simulink model "ExtDem_SelectParameter"  (R2016b)
settings: configuration reference "CodeGenConfigSet" (kept outside this file)
values from neighbouring files (symbols this model uses):
  ExtDem_facFdbk_CUR = Calibration.Parameter    [init_ExtDem_SelectParameter.m]
  ExtDem_facFdbk_CURX = Calibration.Parameter    [init_ExtDem_SelectParameter.m]
  ExtDem_facFdbkLimit_C = Calibration.Parameter    [init_ExtDem_SelectParameter.m]
  ExtDem_facFdbkParSet0_C = Calibration.Parameter    [init_ExtDem_SelectParameter.m]
  ExtDem_facFdbkParSet1_C = Calibration.Parameter    [init_ExtDem_SelectParameter.m]
  ExtDem_facFdbkParSet2_C = Calibration.Parameter    [init_ExtDem_SelectParameter.m]
  ExtDem_facFdbkParSet3_C = Calibration.Parameter    [init_ExtDem_SelectParameter.m]
  ExtDem_facFdbkParSet4_C = Calibration.Parameter    [init_ExtDem_SelectParameter.m]
  ExtDem_facFdbkParSet5_C = Calibration.Parameter    [init_ExtDem_SelectParameter.m]
  ExtDem_facFdbkParSet6_C = Calibration.Parameter    [init_ExtDem_SelectParameter.m]
  ExtDem_facFdbkParSet7_C = Calibration.Parameter    [init_ExtDem_SelectParameter.m]
  ExtDem_facNAvrgPT1CorFac_C = Calibration.Parameter    [init_ExtDem_SelectParameter.m]
  ExtDem_facTrqPT1CorFac_C = Calibration.Parameter    [init_ExtDem_SelectParameter.m]
  ExtDem_KiCorTempFac_MAP = Calibration.Parameter    [init_ExtDem_SelectParameter.m]
  ExtDem_KiCorTempFac_MAPX = Calibration.Parameter    [init_ExtDem_SelectParameter.m]
  ExtDem_KiCorTempFac_MAPY = Calibration.Parameter    [init_ExtDem_SelectParameter.m]
  ExtDem_KiCorTrqFac_MAP = Calibration.Parameter    [init_ExtDem_SelectParameter.m]
  ExtDem_KiCorTrqFac_MAPX = Calibration.Parameter    [init_ExtDem_SelectParameter.m]
  ExtDem_KiCorTrqFac_MAPY = Calibration.Parameter    [init_ExtDem_SelectParameter.m]
  ExtDem_KpCorTempFac_MAP = Calibration.Parameter    [init_ExtDem_SelectParameter.m]
  ExtDem_KpCorTempFac_MAPX = Calibration.Parameter    [init_ExtDem_SelectParameter.m]
  ExtDem_KpCorTempFac_MAPY = Calibration.Parameter    [init_ExtDem_SelectParameter.m]
  ExtDem_KpCorTrqFac_MAP = Calibration.Parameter    [init_ExtDem_SelectParameter.m]
  ExtDem_KpCorTrqFac_MAPX = Calibration.Parameter    [init_ExtDem_SelectParameter.m]
  ExtDem_KpCorTrqFac_MAPY = Calibration.Parameter    [init_ExtDem_SelectParameter.m]
  ExtDem_Par0Cfg_C = Calibration.Parameter    [init_ExtDem_SelectParameter.m]
  ExtDem_Par0dnAccLim_C = Calibration.Parameter    [init_ExtDem_SelectParameter.m]
  ExtDem_Par0dnDeclLim_C = Calibration.Parameter    [init_ExtDem_SelectParameter.m]
  ExtDem_Par0dnDeclLimBrk_C = Calibration.Parameter    [init_ExtDem_SelectParameter.m]
  ExtDem_Par0FacFdbkTrqLosHi_C = Calibration.Parameter    [init_ExtDem_SelectParameter.m]
  ExtDem_Par0FacFdbkTrqLosLo_C = Calibration.Parameter    [init_ExtDem_SelectParameter.m]
  ExtDem_Par0IKi_C = Calibration.Parameter    [init_ExtDem_SelectParameter.m]
  ExtDem_Par0IKiNeg_C = Calibration.Parameter    [init_ExtDem_SelectParameter.m]
  ExtDem_Par0IKiPos_C = Calibration.Parameter    [init_ExtDem_SelectParameter.m]
  ExtDem_Par0InrtVeh_C = Calibration.Parameter    [init_ExtDem_SelectParameter.m]
  ExtDem_Par0nIWinNeg_C = Calibration.Parameter    [init_ExtDem_SelectParameter.m]
  ExtDem_Par0nIWinPos_C = Calibration.Parameter    [init_ExtDem_SelectParameter.m]
  ExtDem_Par0nPWinNeg_C = Calibration.Parameter    [init_ExtDem_SelectParameter.m]
  ExtDem_Par0nPWinPos_C = Calibration.Parameter    [init_ExtDem_SelectParameter.m]
  ExtDem_Par0PKp_C = Calibration.Parameter    [init_ExtDem_SelectParameter.m]
  ExtDem_Par0PKpNeg_C = Calibration.Parameter    [init_ExtDem_SelectParameter.m]
  ExtDem_Par0PKpPos_C = Calibration.Parameter    [init_ExtDem_SelectParameter.m]
  ExtDem_Par0TiFltTrqLosEst_C = Calibration.Parameter    [init_ExtDem_SelectParameter.m]
  ExtDem_Par1Cfg_C = Calibration.Parameter    [init_ExtDem_SelectParameter.m]
  ExtDem_Par1dnAccLim_C = Calibration.Parameter    [init_ExtDem_SelectParameter.m]
  ExtDem_Par1dnDeclLim_C = Calibration.Parameter    [init_ExtDem_SelectParameter.m]
  ExtDem_Par1dnDeclLimBrk_C = Calibration.Parameter    [init_ExtDem_SelectParameter.m]
  ExtDem_Par1FacFdbkTrqLosHi_C = Calibration.Parameter    [init_ExtDem_SelectParameter.m]
  ExtDem_Par1FacFdbkTrqLosLo_C = Calibration.Parameter    [init_ExtDem_SelectParameter.m]
  ExtDem_Par1IKi_C = Calibration.Parameter    [init_ExtDem_SelectParameter.m]
  ExtDem_Par1IKiNeg_C = Calibration.Parameter    [init_ExtDem_SelectParameter.m]
  ExtDem_Par1IKiPos_C = Calibration.Parameter    [init_ExtDem_SelectParameter.m]
  ExtDem_Par1InrtVeh_C = Calibration.Parameter    [init_ExtDem_SelectParameter.m]
  ExtDem_Par1nIWinNeg_C = Calibration.Parameter    [init_ExtDem_SelectParameter.m]
  ExtDem_Par1nIWinPos_C = Calibration.Parameter    [init_ExtDem_SelectParameter.m]
  ExtDem_Par1nPWinNeg_C = Calibration.Parameter    [init_ExtDem_SelectParameter.m]
  ExtDem_Par1nPWinPos_C = Calibration.Parameter    [init_ExtDem_SelectParameter.m]
  ExtDem_Par1PKp_C = Calibration.Parameter    [init_ExtDem_SelectParameter.m]
  ExtDem_Par1PKpNeg_C = Calibration.Parameter    [init_ExtDem_SelectParameter.m]
  ExtDem_Par1PKpPos_C = Calibration.Parameter    [init_ExtDem_SelectParameter.m]
  ExtDem_Par1TiFltTrqLosEst_C = Calibration.Parameter    [init_ExtDem_SelectParameter.m]
  ExtDem_Par2Cfg_C = Calibration.Parameter    [init_ExtDem_SelectParameter.m]
  ExtDem_Par2dnAccLim_C = Calibration.Parameter    [init_ExtDem_SelectParameter.m]
  ExtDem_Par2dnDeclLim_C = Calibration.Parameter    [init_ExtDem_SelectParameter.m]
  ExtDem_Par2dnDeclLimBrk_C = Calibration.Parameter    [init_ExtDem_SelectParameter.m]
  ExtDem_Par2FacFdbkTrqLosHi_C = Calibration.Parameter    [init_ExtDem_SelectParameter.m]
  ExtDem_Par2FacFdbkTrqLosLo_C = Calibration.Parameter    [init_ExtDem_SelectParameter.m]
  ExtDem_Par2IKi_C = Calibration.Parameter    [init_ExtDem_SelectParameter.m]
  ExtDem_Par2IKiNeg_C = Calibration.Parameter    [init_ExtDem_SelectParameter.m]
  ExtDem_Par2IKiPos_C = Calibration.Parameter    [init_ExtDem_SelectParameter.m]
  ExtDem_Par2InrtVeh_C = Calibration.Parameter    [init_ExtDem_SelectParameter.m]
  ExtDem_Par2nIWinNeg_C = Calibration.Parameter    [init_ExtDem_SelectParameter.m]
  ExtDem_Par2nIWinPos_C = Calibration.Parameter    [init_ExtDem_SelectParameter.m]
  ExtDem_Par2nPWinNeg_C = Calibration.Parameter    [init_ExtDem_SelectParameter.m]
  ExtDem_Par2nPWinPos_C = Calibration.Parameter    [init_ExtDem_SelectParameter.m]
  ExtDem_Par2PKp_C = Calibration.Parameter    [init_ExtDem_SelectParameter.m]
  ExtDem_Par2PKpNeg_C = Calibration.Parameter    [init_ExtDem_SelectParameter.m]
  ExtDem_Par2PKpPos_C = Calibration.Parameter    [init_ExtDem_SelectParameter.m]
  ExtDem_Par2TiFltTrqLosEst_C = Calibration.Parameter    [init_ExtDem_SelectParameter.m]
  ExtDem_Par3Cfg_C = Calibration.Parameter    [init_ExtDem_SelectParameter.m]
  ExtDem_Par3dnAccLim_C = Calibration.Parameter    [init_ExtDem_SelectParameter.m]
  ExtDem_Par3dnDeclLim_C = Calibration.Parameter    [init_ExtDem_SelectParameter.m]
  ExtDem_Par3dnDeclLimBrk_C = Calibration.Parameter    [init_ExtDem_SelectParameter.m]
  ExtDem_Par3FacFdbkTrqLosHi_C = Calibration.Parameter    [init_ExtDem_SelectParameter.m]
  ExtDem_Par3FacFdbkTrqLosLo_C = Calibration.Parameter    [init_ExtDem_SelectParameter.m]
  ExtDem_Par3IKi_C = Calibration.Parameter    [init_ExtDem_SelectParameter.m]
  ExtDem_Par3IKiNeg_C = Calibration.Parameter    [init_ExtDem_SelectParameter.m]
  ExtDem_Par3IKiPos_C = Calibration.Parameter    [init_ExtDem_SelectParameter.m]
  ExtDem_Par3InrtVeh_C = Calibration.Parameter    [init_ExtDem_SelectParameter.m]
  ExtDem_Par3nIWinNeg_C = Calibration.Parameter    [init_ExtDem_SelectParameter.m]
  ExtDem_Par3nIWinPos_C = Calibration.Parameter    [init_ExtDem_SelectParameter.m]
  ExtDem_Par3nPWinNeg_C = Calibration.Parameter    [init_ExtDem_SelectParameter.m]
  ExtDem_Par3nPWinPos_C = Calibration.Parameter    [init_ExtDem_SelectParameter.m]
  ExtDem_Par3PKp_C = Calibration.Parameter    [init_ExtDem_SelectParameter.m]
  ExtDem_Par3PKpNeg_C = Calibration.Parameter    [init_ExtDem_SelectParameter.m]
  ExtDem_Par3PKpPos_C = Calibration.Parameter    [init_ExtDem_SelectParameter.m]
  ExtDem_Par3TiFltTrqLosEst_C = Calibration.Parameter    [init_ExtDem_SelectParameter.m]
  ExtDem_Par4Cfg_C = Calibration.Parameter    [init_ExtDem_SelectParameter.m]
  ExtDem_Par4dnAccLim_C = Calibration.Parameter    [init_ExtDem_SelectParameter.m]
  ExtDem_Par4dnDeclLim_C = Calibration.Parameter    [init_ExtDem_SelectParameter.m]
  ExtDem_Par4dnDeclLimBrk_C = Calibration.Parameter    [init_ExtDem_SelectParameter.m]
  ExtDem_Par4FacFdbkTrqLosHi_C = Calibration.Parameter    [init_ExtDem_SelectParameter.m]
  ExtDem_Par4FacFdbkTrqLosLo_C = Calibration.Parameter    [init_ExtDem_SelectParameter.m]
  ExtDem_Par4IKi_C = Calibration.Parameter    [init_ExtDem_SelectParameter.m]
  ExtDem_Par4IKiNeg_C = Calibration.Parameter    [init_ExtDem_SelectParameter.m]
  ExtDem_Par4IKiPos_C = Calibration.Parameter    [init_ExtDem_SelectParameter.m]
  ExtDem_Par4InrtVeh_C = Calibration.Parameter    [init_ExtDem_SelectParameter.m]
  ExtDem_Par4nIWinNeg_C = Calibration.Parameter    [init_ExtDem_SelectParameter.m]
  ExtDem_Par4nIWinPos_C = Calibration.Parameter    [init_ExtDem_SelectParameter.m]
  ExtDem_Par4nPWinNeg_C = Calibration.Parameter    [init_ExtDem_SelectParameter.m]
  ExtDem_Par4nPWinPos_C = Calibration.Parameter    [init_ExtDem_SelectParameter.m]
  ExtDem_Par4PKp_C = Calibration.Parameter    [init_ExtDem_SelectParameter.m]
  ExtDem_Par4PKpNeg_C = Calibration.Parameter    [init_ExtDem_SelectParameter.m]
  ExtDem_Par4PKpPos_C = Calibration.Parameter    [init_ExtDem_SelectParameter.m]
  ExtDem_Par4TiFltTrqLosEst_C = Calibration.Parameter    [init_ExtDem_SelectParameter.m]
  ExtDem_Par5Cfg_C = Calibration.Parameter    [init_ExtDem_SelectParameter.m]
  ExtDem_Par5dnAccLim_C = Calibration.Parameter    [init_ExtDem_SelectParameter.m]
  ExtDem_Par5dnDeclLim_C = Calibration.Parameter    [init_ExtDem_SelectParameter.m]
  ExtDem_Par5dnDeclLimBrk_C = Calibration.Parameter    [init_ExtDem_SelectParameter.m]
  ExtDem_Par5FacFdbkTrqLosHi_C = Calibration.Parameter    [init_ExtDem_SelectParameter.m]
  ... (+56 more)
libraries: CXLib x7
(part 2 of 2)

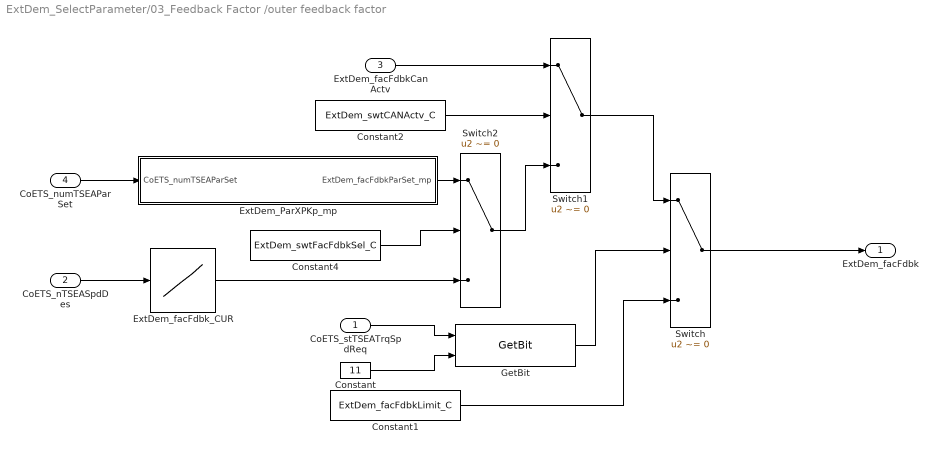
== system ExtDem_SelectParameter/03_Feedback Factor /outer feedback factor  ==
  CoETS_stTSEATrqSpdReq : Inport  Description=Status of information about torque and speed intervention  OutMin=0  OutMax=65535  OutDataTypeStr=State_uint16
  CoETS_nTSEASpdDes : Inport  Tag=rpm  Description=The desired/control engine speed requested from TSC1 CAN messages  Port=2  OutMin=0  OutMax=6000  OutDataTypeStr=EngSpeed_rpm
  ExtDem_facFdbkCanActv : Inport  Tag=rpm/Nm  Description=External intervention feedback factor from CAN  Port=3  OutMin=-20  OutMax=20  OutDataTypeStr=FdbkNm2rpm_rpm_Nm
  CoETS_numTSEAParSet : Inport  Description=Number of requested parameter set for Engine speed governor  Port=4  OutMin=0  OutMax=255  OutDataTypeStr=State_uint8
  Constant : Constant  Value=11  OutDataTypeStr=uint8
  Constant1 : Constant  Value=ExtDem_facFdbkLimit_C
  Constant2 : Constant  Value=ExtDem_swtCANActv_C
  Constant4 : Constant  Value=ExtDem_swtFacFdbkSel_C
  ExtDem_ParXPKp_mp : Subsystem
  ExtDem_facFdbk_CUR : Lookup_n-D  NumberOfTableDimensions=1  BreakpointsForDimension1=ExtDem_facFdbk_CURX  BeginIndexSearchUsingPreviousIndexResult=on  Table=ExtDem_facFdbk_CUR  ExtrapMethod=Clip  UseLastTableValue=on  InternalRulePriority=Speed  OutDataTypeStr=Inherit: Inherit from 'Table data'  RndMeth=Simplest  InputSameDT=on
  GetBit : CXLib/GetBit  dataTypeString=uint16  dataLength=0
      settings: AttributesFormatString=Get bit from %<dataTypeString>
  Switch : Switch  Criteria=u2 ~= 0
  Switch1 : Switch  Criteria=u2 ~= 0
  Switch2 : Switch  Criteria=u2 ~= 0
  ExtDem_facFdbk : Outport  Tag=rpm/Nm  Description=External intervention feedback factor  OutMin=-20  OutMax=20  OutDataTypeStr=FdbkNm2rpm_rpm_Nm
  wires:
  CoETS_stTSEATrqSpdReq/1 -> GetBit/1
  Constant/1 -> GetBit/2
  GetBit/1 -> Switch/2
  Switch1/1 -> Switch/1
  Constant2/1 -> Switch1/2
  Constant4/1 -> Switch2/2
  ExtDem_ParXPKp_mp/1(ExtDem_facFdbkParSet_mp) -> Switch2/1
  CoETS_numTSEAParSet/1 -> ExtDem_ParXPKp_mp/1(CoETS_numTSEAParSet)
  CoETS_nTSEASpdDes/1 -> ExtDem_facFdbk_CUR/1
  Switch/1 -> ExtDem_facFdbk/1
  Constant1/1 -> Switch/3
  ExtDem_facFdbkCanActv/1 -> Switch1/1
  Switch2/1 -> Switch1/3
  ExtDem_facFdbk_CUR/1 -> Switch2/3

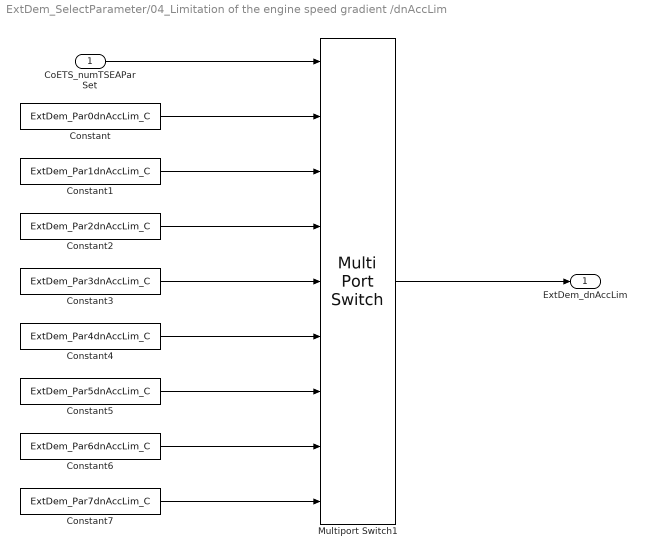
== system ExtDem_SelectParameter/04_Limitation of the engine speed gradient /dnAccLim ==
  CoETS_numTSEAParSet : Inport  Description=Number of requested parameter set for Engine speed governor  OutMin=0  OutMax=255  OutDataTypeStr=State_uint8
  Constant : Constant  Value=ExtDem_Par0dnAccLim_C
  Constant1 : Constant  Value=ExtDem_Par1dnAccLim_C
  Constant2 : Constant  Value=ExtDem_Par2dnAccLim_C
  Constant3 : Constant  Value=ExtDem_Par3dnAccLim_C
  Constant4 : Constant  Value=ExtDem_Par4dnAccLim_C
  Constant5 : Constant  Value=ExtDem_Par5dnAccLim_C
  Constant6 : Constant  Value=ExtDem_Par6dnAccLim_C
  Constant7 : Constant  Value=ExtDem_Par7dnAccLim_C
  Multiport Switch1 : MultiPortSwitch  DataPortOrder=Zero-based contiguous  Inputs=8
  ExtDem_dnAccLim : Outport  Tag=rpm/s  Description=Maximum permissible acceleration (Engine speed)  OutMin=-12000  OutMax=12000  OutDataTypeStr=EngSpeed_rpm_s
  wires:
  Multiport Switch1/1 -> ExtDem_dnAccLim/1
  CoETS_numTSEAParSet/1 -> Multiport Switch1/1
  Constant/1 -> Multiport Switch1/2
  Constant1/1 -> Multiport Switch1/3
  Constant2/1 -> Multiport Switch1/4
  Constant3/1 -> Multiport Switch1/5
  Constant4/1 -> Multiport Switch1/6
  Constant5/1 -> Multiport Switch1/7
  Constant6/1 -> Multiport Switch1/8
  Constant7/1 -> Multiport Switch1/9

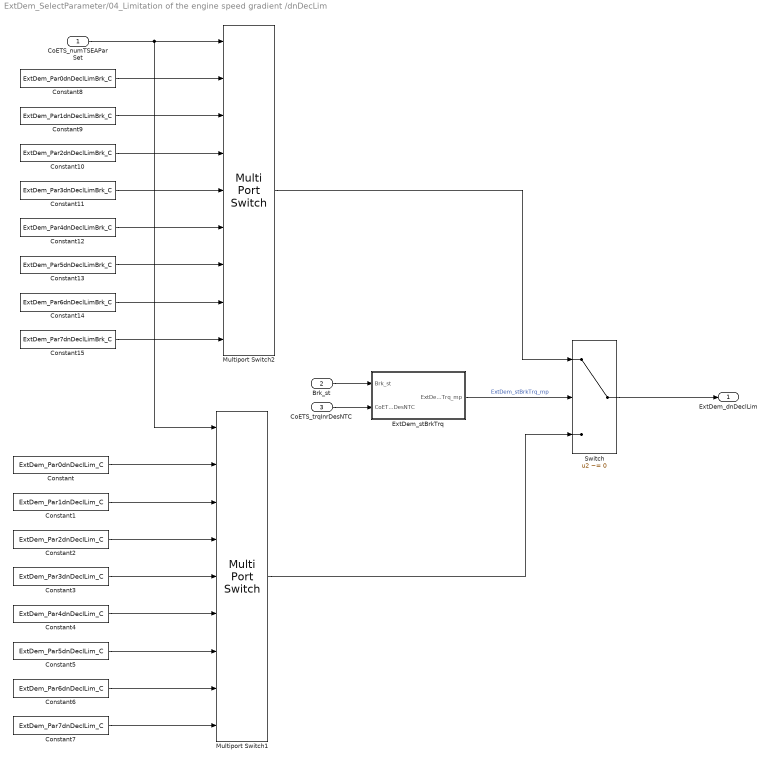
== system ExtDem_SelectParameter/04_Limitation of the engine speed gradient /dnDecLim ==
  CoETS_numTSEAParSet : Inport  Description=Number of requested parameter set for Engine speed governor  OutMin=0  OutMax=255  OutDataTypeStr=State_uint8
  Brk_st : Inport  Description=Brake switch state  Port=2  OutMin=0  OutMax=255  OutDataTypeStr=State_uint8
  CoETS_trqInrDesNTC : Inport  Tag=Nm  Description=Additional desired engine friction Nm  Port=3  OutMin=-3276  OutMax=3276  OutDataTypeStr=Trq_Nm
  Constant : Constant  Value=ExtDem_Par0dnDeclLim_C
  Constant1 : Constant  Value=ExtDem_Par1dnDeclLim_C
  Constant10 : Constant  Value=ExtDem_Par2dnDeclLimBrk_C
  Constant11 : Constant  Value=ExtDem_Par3dnDeclLimBrk_C
  Constant12 : Constant  Value=ExtDem_Par4dnDeclLimBrk_C
  Constant13 : Constant  Value=ExtDem_Par5dnDeclLimBrk_C
  Constant14 : Constant  Value=ExtDem_Par6dnDeclLimBrk_C
  Constant15 : Constant  Value=ExtDem_Par7dnDeclLimBrk_C
  Constant2 : Constant  Value=ExtDem_Par2dnDeclLim_C
  Constant3 : Constant  Value=ExtDem_Par3dnDeclLim_C
  Constant4 : Constant  Value=ExtDem_Par4dnDeclLim_C
  Constant5 : Constant  Value=ExtDem_Par5dnDeclLim_C
  Constant6 : Constant  Value=ExtDem_Par6dnDeclLim_C
  Constant7 : Constant  Value=ExtDem_Par7dnDeclLim_C
  Constant8 : Constant  Value=ExtDem_Par0dnDeclLimBrk_C
  Constant9 : Constant  Value=ExtDem_Par1dnDeclLimBrk_C
  ExtDem_stBrkTrq : Subsystem
  Multiport Switch1 : MultiPortSwitch  DataPortOrder=Zero-based contiguous  Inputs=8
  Multiport Switch2 : MultiPortSwitch  DataPortOrder=Zero-based contiguous  Inputs=8
  Switch : Switch  Criteria=u2 ~= 0
  ExtDem_dnDeclLim : Outport  Tag=rpm/s  Description=Maximum permissible deceleration (Engine speed)  OutMin=-12000  OutMax=12000  OutDataTypeStr=EngSpeed_rpm_s
  wires:
  Constant7/1 -> Multiport Switch1/9
  Constant6/1 -> Multiport Switch1/8
  Constant5/1 -> Multiport Switch1/7
  Constant4/1 -> Multiport Switch1/6
  Constant3/1 -> Multiport Switch1/5
  Constant2/1 -> Multiport Switch1/4
  Constant1/1 -> Multiport Switch1/3
  Constant/1 -> Multiport Switch1/2
  Switch/1 -> ExtDem_dnDeclLim/1
  Constant15/1 -> Multiport Switch2/9
  Constant14/1 -> Multiport Switch2/8
  Constant13/1 -> Multiport Switch2/7
  Constant12/1 -> Multiport Switch2/6
  Constant11/1 -> Multiport Switch2/5
  Constant10/1 -> Multiport Switch2/4
  Constant9/1 -> Multiport Switch2/3
  Constant8/1 -> Multiport Switch2/2
  CoETS_numTSEAParSet/1 -> Multiport Switch1/1, Multiport Switch2/1
  Multiport Switch2/1 -> Switch/1
  Multiport Switch1/1 -> Switch/3
  Brk_st/1 -> ExtDem_stBrkTrq/1(Brk_st)
  CoETS_trqInrDesNTC/1 -> ExtDem_stBrkTrq/2(CoETS_trqInrDesNTC)
  ExtDem_stBrkTrq/1(ExtDem_stBrkTrq_mp) -> Switch/2  "ExtDem_stBrkTrq_mp"

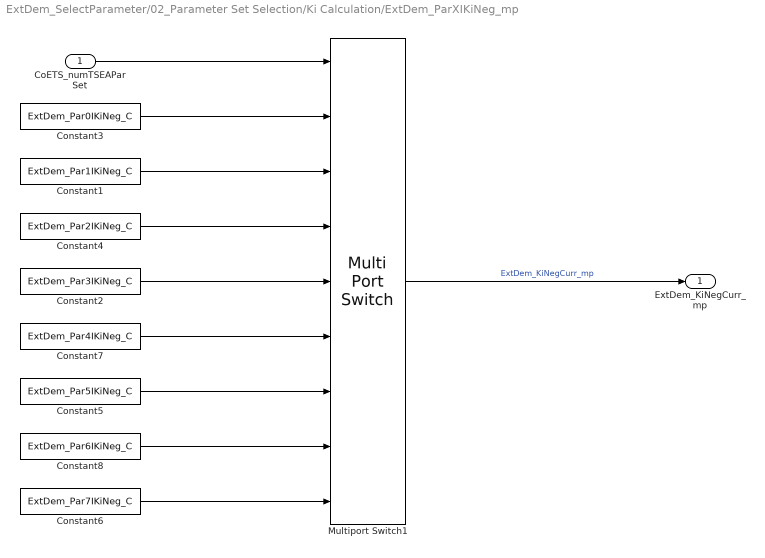
== system ExtDem_SelectParameter/02_Parameter Set Selection/Ki Calculation/ExtDem_ParXIKiNeg_mp ==
  CoETS_numTSEAParSet : Inport  Description=Number of requested parameter set for Engine speed governor  OutMin=0  OutMax=255  OutDataTypeStr=State_uint8
  Constant1 : Constant  Value=ExtDem_Par1IKiNeg_C
  Constant2 : Constant  Value=ExtDem_Par3IKiNeg_C
  Constant3 : Constant  Value=ExtDem_Par0IKiNeg_C
  Constant4 : Constant  Value=ExtDem_Par2IKiNeg_C
  Constant5 : Constant  Value=ExtDem_Par5IKiNeg_C
  Constant6 : Constant  Value=ExtDem_Par7IKiNeg_C
  Constant7 : Constant  Value=ExtDem_Par4IKiNeg_C
  Constant8 : Constant  Value=ExtDem_Par6IKiNeg_C
  Multiport Switch1 : MultiPortSwitch  DataPortOrder=Zero-based contiguous  Inputs=8
  ExtDem_KiNegCurr_mp : Outport
  wires:
  CoETS_numTSEAParSet/1 -> Multiport Switch1/1
  Constant6/1 -> Multiport Switch1/9
  Constant8/1 -> Multiport Switch1/8
  Constant5/1 -> Multiport Switch1/7
  Constant7/1 -> Multiport Switch1/6
  Constant2/1 -> Multiport Switch1/5
  Constant4/1 -> Multiport Switch1/4
  Constant1/1 -> Multiport Switch1/3
  Constant3/1 -> Multiport Switch1/2
  Multiport Switch1/1 -> ExtDem_KiNegCurr_mp/1  "ExtDem_KiNegCurr_mp"

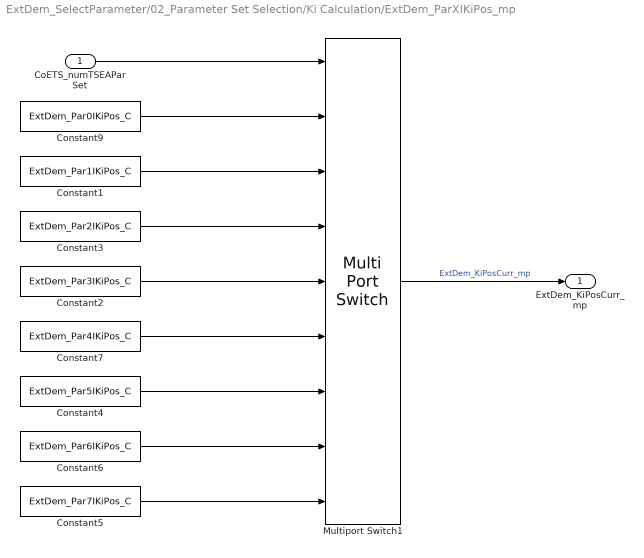
== system ExtDem_SelectParameter/02_Parameter Set Selection/Ki Calculation/ExtDem_ParXIKiPos_mp ==
  CoETS_numTSEAParSet : Inport  Description=Number of requested parameter set for Engine speed governor  OutMin=0  OutMax=255  OutDataTypeStr=State_uint8
  Constant1 : Constant  Value=ExtDem_Par1IKiPos_C
  Constant2 : Constant  Value=ExtDem_Par3IKiPos_C
  Constant3 : Constant  Value=ExtDem_Par2IKiPos_C
  Constant4 : Constant  Value=ExtDem_Par5IKiPos_C
  Constant5 : Constant  Value=ExtDem_Par7IKiPos_C
  Constant6 : Constant  Value=ExtDem_Par6IKiPos_C
  Constant7 : Constant  Value=ExtDem_Par4IKiPos_C
  Constant9 : Constant  Value=ExtDem_Par0IKiPos_C
  Multiport Switch1 : MultiPortSwitch  DataPortOrder=Zero-based contiguous  Inputs=8
  ExtDem_KiPosCurr_mp : Outport
  wires:
  Constant9/1 -> Multiport Switch1/2
  Constant1/1 -> Multiport Switch1/3
  Constant3/1 -> Multiport Switch1/4
  Constant2/1 -> Multiport Switch1/5
  Constant7/1 -> Multiport Switch1/6
  Constant4/1 -> Multiport Switch1/7
  Constant6/1 -> Multiport Switch1/8
  Constant5/1 -> Multiport Switch1/9
  CoETS_numTSEAParSet/1 -> Multiport Switch1/1
  Multiport Switch1/1 -> ExtDem_KiPosCurr_mp/1  "ExtDem_KiPosCurr_mp"

== system ExtDem_SelectParameter/02_Parameter Set Selection/Ki Calculation/ExtDem_ParXIKi_mp ==
  CoETS_numTSEAParSet : Inport  Description=Number of requested parameter set for Engine speed governor  OutMin=0  OutMax=255  OutDataTypeStr=State_uint8
  Constant1 : Constant  Value=ExtDem_Par0IKi_C
  Constant2 : Constant  Value=ExtDem_Par1IKi_C
  Constant3 : Constant  Value=ExtDem_Par2IKi_C
  Constant4 : Constant  Value=ExtDem_Par3IKi_C
  Constant5 : Constant  Value=ExtDem_Par4IKi_C
  Constant6 : Constant  Value=ExtDem_Par5IKi_C
  Constant7 : Constant  Value=ExtDem_Par6IKi_C
  Constant8 : Constant  Value=ExtDem_Par7IKi_C
  Multiport Switch1 : MultiPortSwitch  DataPortOrder=Zero-based contiguous  Inputs=8
  ExtDem_KiCurr_mp : Outport
  wires:
  Multiport Switch1/1 -> ExtDem_KiCurr_mp/1  "ExtDem_KiCurr_mp"
  CoETS_numTSEAParSet/1 -> Multiport Switch1/1
  Constant8/1 -> Multiport Switch1/9
  Constant7/1 -> Multiport Switch1/8
  Constant6/1 -> Multiport Switch1/7
  Constant5/1 -> Multiport Switch1/6
  Constant4/1 -> Multiport Switch1/5
  Constant3/1 -> Multiport Switch1/4
  Constant2/1 -> Multiport Switch1/3
  Constant1/1 -> Multiport Switch1/2

== system ExtDem_SelectParameter/02_Parameter Set Selection/Ki Calculation/ExtDem_ParXnIWinNeg_mp ==
  CoETS_numTSEAParSet : Inport  Description=Number of requested parameter set for Engine speed governor  OutMin=0  OutMax=255  OutDataTypeStr=State_uint8
  Constant1 : Constant  Value=ExtDem_Par1nIWinNeg_C
  Constant2 : Constant  Value=ExtDem_Par2nIWinNeg_C
  Constant3 : Constant  Value=ExtDem_Par3nIWinNeg_C
  Constant4 : Constant  Value=ExtDem_Par4nIWinNeg_C
  Constant5 : Constant  Value=ExtDem_Par0nIWinNeg_C
  Constant6 : Constant  Value=ExtDem_Par5nIWinNeg_C
  Constant7 : Constant  Value=ExtDem_Par6nIWinNeg_C
  Constant8 : Constant  Value=ExtDem_Par7nIWinNeg_C
  Multiport Switch1 : MultiPortSwitch  DataPortOrder=Zero-based contiguous  Inputs=8
  ExtDem_IWinNegCurr : Outport
  wires:
  Multiport Switch1/1 -> ExtDem_IWinNegCurr/1  "ExtDem_IWinNegCurr"
  CoETS_numTSEAParSet/1 -> Multiport Switch1/1
  Constant8/1 -> Multiport Switch1/9
  Constant7/1 -> Multiport Switch1/8
  Constant6/1 -> Multiport Switch1/7
  Constant4/1 -> Multiport Switch1/6
  Constant3/1 -> Multiport Switch1/5
  Constant2/1 -> Multiport Switch1/4
  Constant1/1 -> Multiport Switch1/3
  Constant5/1 -> Multiport Switch1/2

== system ExtDem_SelectParameter/02_Parameter Set Selection/Ki Calculation/ExtDem_ParXnIWinPos_mp ==
  CoETS_numTSEAParSet : Inport  Description=Number of requested parameter set for Engine speed governor  OutMin=0  OutMax=255  OutDataTypeStr=State_uint8
  Constant1 : Constant  Value=ExtDem_Par1nIWinPos_C
  Constant2 : Constant  Value=ExtDem_Par2nIWinPos_C
  Constant3 : Constant  Value=ExtDem_Par3nIWinPos_C
  Constant4 : Constant  Value=ExtDem_Par0nIWinPos_C
  Constant5 : Constant  Value=ExtDem_Par4nIWinPos_C
  Constant6 : Constant  Value=ExtDem_Par5nIWinPos_C
  Constant7 : Constant  Value=ExtDem_Par6nIWinPos_C
  Constant8 : Constant  Value=ExtDem_Par7nIWinPos_C
  Multiport Switch1 : MultiPortSwitch  DataPortOrder=Zero-based contiguous  Inputs=8
  ExtDem_IWinPosCurr : Outport
  wires:
  Constant4/1 -> Multiport Switch1/2
  Constant1/1 -> Multiport Switch1/3
  Constant2/1 -> Multiport Switch1/4
  Constant3/1 -> Multiport Switch1/5
  Constant5/1 -> Multiport Switch1/6
  Constant6/1 -> Multiport Switch1/7
  Constant7/1 -> Multiport Switch1/8
  Constant8/1 -> Multiport Switch1/9
  CoETS_numTSEAParSet/1 -> Multiport Switch1/1
  Multiport Switch1/1 -> ExtDem_IWinPosCurr/1  "ExtDem_IWinPosCurr"

== system ExtDem_SelectParameter/02_Parameter Set Selection/Kp Calculation /ExtDem_PWinNeg ==
  CoETS_numTSEAParSet : Inport  Description=Number of requested parameter set for Engine speed governor  OutMin=0  OutMax=255  OutDataTypeStr=State_uint8
  Constant1 : Constant  Value=ExtDem_Par1nPWinNeg_C
  Constant2 : Constant  Value=ExtDem_Par2nPWinNeg_C
  Constant3 : Constant  Value=ExtDem_Par3nPWinNeg_C
  Constant4 : Constant  Value=ExtDem_Par4nPWinNeg_C
  Constant5 : Constant  Value=ExtDem_Par0nPWinNeg_C
  Constant6 : Constant  Value=ExtDem_Par5nPWinNeg_C
  Constant7 : Constant  Value=ExtDem_Par6nPWinNeg_C
  Constant8 : Constant  Value=ExtDem_Par7nPWinNeg_C
  Multiport Switch1 : MultiPortSwitch  DataPortOrder=Zero-based contiguous  Inputs=8
  ExtDem_PWinNegCurr : Outport
  wires:
  Constant5/1 -> Multiport Switch1/2
  Constant1/1 -> Multiport Switch1/3
  Constant2/1 -> Multiport Switch1/4
  Constant3/1 -> Multiport Switch1/5
  Constant4/1 -> Multiport Switch1/6
  Constant6/1 -> Multiport Switch1/7
  Constant7/1 -> Multiport Switch1/8
  Constant8/1 -> Multiport Switch1/9
  CoETS_numTSEAParSet/1 -> Multiport Switch1/1
  Multiport Switch1/1 -> ExtDem_PWinNegCurr/1  "ExtDem_PWinNegCurr"

== system ExtDem_SelectParameter/02_Parameter Set Selection/Kp Calculation /ExtDem_PWinPos ==
  CoETS_numTSEAParSet : Inport  Description=Number of requested parameter set for Engine speed governor  OutMin=0  OutMax=255  OutDataTypeStr=State_uint8
  Constant1 : Constant  Value=ExtDem_Par1nPWinPos_C
  Constant2 : Constant  Value=ExtDem_Par2nPWinPos_C
  Constant3 : Constant  Value=ExtDem_Par3nPWinPos_C
  Constant4 : Constant  Value=ExtDem_Par0nPWinPos_C
  Constant5 : Constant  Value=ExtDem_Par4nPWinPos_C
  Constant6 : Constant  Value=ExtDem_Par5nPWinPos_C
  Constant7 : Constant  Value=ExtDem_Par6nPWinPos_C
  Constant8 : Constant  Value=ExtDem_Par7nPWinPos_C
  Multiport Switch1 : MultiPortSwitch  DataPortOrder=Zero-based contiguous  Inputs=8
  ExtDem_PWinPosCurr : Outport
  wires:
  Multiport Switch1/1 -> ExtDem_PWinPosCurr/1  "ExtDem_PWinPosCurr"
  CoETS_numTSEAParSet/1 -> Multiport Switch1/1
  Constant8/1 -> Multiport Switch1/9
  Constant7/1 -> Multiport Switch1/8
  Constant6/1 -> Multiport Switch1/7
  Constant5/1 -> Multiport Switch1/6
  Constant3/1 -> Multiport Switch1/5
  Constant2/1 -> Multiport Switch1/4
  Constant1/1 -> Multiport Switch1/3
  Constant4/1 -> Multiport Switch1/2

== system ExtDem_SelectParameter/02_Parameter Set Selection/Kp Calculation /ExtDem_ParXPKpNeg_mp ==
  CoETS_numTSEAParSet : Inport  Description=Number of requested parameter set for Engine speed governor  OutMin=0  OutMax=255  OutDataTypeStr=State_uint8
  Constant1 : Constant  Value=ExtDem_Par1PKpNeg_C
  Constant2 : Constant  Value=ExtDem_Par3PKpNeg_C
  Constant3 : Constant  Value=ExtDem_Par0PKpNeg_C
  Constant4 : Constant  Value=ExtDem_Par2PKpNeg_C
  Constant5 : Constant  Value=ExtDem_Par5PKpNeg_C
  Constant6 : Constant  Value=ExtDem_Par7PKpNeg_C
  Constant7 : Constant  Value=ExtDem_Par4PKpNeg_C
  Constant8 : Constant  Value=ExtDem_Par6PKpNeg_C
  Multiport Switch1 : MultiPortSwitch  DataPortOrder=Zero-based contiguous  Inputs=8
  ExtDem_KpNegCurr_mp : Outport
  wires:
  Constant3/1 -> Multiport Switch1/2
  Constant1/1 -> Multiport Switch1/3
  Constant4/1 -> Multiport Switch1/4
  Constant2/1 -> Multiport Switch1/5
  Constant7/1 -> Multiport Switch1/6
  Constant5/1 -> Multiport Switch1/7
  Constant8/1 -> Multiport Switch1/8
  Constant6/1 -> Multiport Switch1/9
  CoETS_numTSEAParSet/1 -> Multiport Switch1/1
  Multiport Switch1/1 -> ExtDem_KpNegCurr_mp/1  "ExtDem_KpNegCurr_mp"

== system ExtDem_SelectParameter/02_Parameter Set Selection/Kp Calculation /ExtDem_ParXPKpPos_mp ==
  CoETS_numTSEAParSet : Inport  Description=Number of requested parameter set for Engine speed governor  OutMin=0  OutMax=255  OutDataTypeStr=State_uint8
  Constant1 : Constant  Value=ExtDem_Par1PKpPos_C
  Constant2 : Constant  Value=ExtDem_Par3PKpPos_C
  Constant3 : Constant  Value=ExtDem_Par2PKpPos_C
  Constant4 : Constant  Value=ExtDem_Par5PKpPos_C
  Constant5 : Constant  Value=ExtDem_Par7PKpPos_C
  Constant6 : Constant  Value=ExtDem_Par6PKpPos_C
  Constant7 : Constant  Value=ExtDem_Par4PKpPos_C
  Constant9 : Constant  Value=ExtDem_Par0PKpPos_C
  Multiport Switch1 : MultiPortSwitch  DataPortOrder=Zero-based contiguous  Inputs=8
  ExtDem_KpPosCurr_mp : Outport
  wires:
  Multiport Switch1/1 -> ExtDem_KpPosCurr_mp/1  "ExtDem_KpPosCurr_mp"
  CoETS_numTSEAParSet/1 -> Multiport Switch1/1
  Constant5/1 -> Multiport Switch1/9
  Constant6/1 -> Multiport Switch1/8
  Constant4/1 -> Multiport Switch1/7
  Constant7/1 -> Multiport Switch1/6
  Constant2/1 -> Multiport Switch1/5
  Constant3/1 -> Multiport Switch1/4
  Constant1/1 -> Multiport Switch1/3
  Constant9/1 -> Multiport Switch1/2

== system ExtDem_SelectParameter/02_Parameter Set Selection/Kp Calculation /ExtDem_ParXPKp_mp ==
  CoETS_numTSEAParSet : Inport  Description=Number of requested parameter set for Engine speed governor  OutMin=0  OutMax=255  OutDataTypeStr=State_uint8
  Constant1 : Constant  Value=ExtDem_Par0PKp_C
  Constant2 : Constant  Value=ExtDem_Par1PKp_C
  Constant3 : Constant  Value=ExtDem_Par2PKp_C
  Constant4 : Constant  Value=ExtDem_Par3PKp_C
  Constant5 : Constant  Value=ExtDem_Par4PKp_C
  Constant6 : Constant  Value=ExtDem_Par5PKp_C
  Constant7 : Constant  Value=ExtDem_Par6PKp_C
  Constant8 : Constant  Value=ExtDem_Par7PKp_C
  Multiport Switch1 : MultiPortSwitch  DataPortOrder=Zero-based contiguous  Inputs=8
  ExtDem_KpCurr_mp : Outport
  wires:
  Constant1/1 -> Multiport Switch1/2
  Constant2/1 -> Multiport Switch1/3
  Constant3/1 -> Multiport Switch1/4
  Constant4/1 -> Multiport Switch1/5
  Constant5/1 -> Multiport Switch1/6
  Constant6/1 -> Multiport Switch1/7
  Constant7/1 -> Multiport Switch1/8
  Constant8/1 -> Multiport Switch1/9
  CoETS_numTSEAParSet/1 -> Multiport Switch1/1
  Multiport Switch1/1 -> ExtDem_KpCurr_mp/1  "ExtDem_KpCurr_mp"

== system ExtDem_SelectParameter/03_Feedback Factor / inner feedback factors /InrtVehCurr ==
  CoETS_numTSEAParSet : Inport  Description=Number of requested parameter set for Engine speed governor  OutMin=0  OutMax=255  OutDataTypeStr=State_uint8
  Constant : Constant  Value=ExtDem_Par0InrtVeh_C
  Constant1 : Constant  Value=ExtDem_Par1InrtVeh_C
  Constant2 : Constant  Value=ExtDem_Par2InrtVeh_C
  Constant3 : Constant  Value=ExtDem_Par3InrtVeh_C
  Constant4 : Constant  Value=ExtDem_Par4InrtVeh_C
  Constant5 : Constant  Value=ExtDem_Par5InrtVeh_C
  Constant6 : Constant  Value=ExtDem_Par6InrtVeh_C
  Constant7 : Constant  Value=ExtDem_Par7InrtVeh_C
  Multiport Switch1 : MultiPortSwitch  DataPortOrder=Zero-based contiguous  Inputs=8
  ExtDem_InrtVehCurr : Outport  Tag=Nm/(rpm/s)  Description=Mass inirtia for EISGov torque loss estimation  OutMin=-50  OutMax=50  OutDataTypeStr=HLSDem_Inrt
  wires:
  Constant/1 -> Multiport Switch1/2
  Constant1/1 -> Multiport Switch1/3
  Constant2/1 -> Multiport Switch1/4
  Constant3/1 -> Multiport Switch1/5
  Constant4/1 -> Multiport Switch1/6
  Constant5/1 -> Multiport Switch1/7
  Constant6/1 -> Multiport Switch1/8
  Constant7/1 -> Multiport Switch1/9
  CoETS_numTSEAParSet/1 -> Multiport Switch1/1
  Multiport Switch1/1 -> ExtDem_InrtVehCurr/1

== system ExtDem_SelectParameter/03_Feedback Factor / inner feedback factors /facFdbkTrqLosHi ==
  CoETS_numTSEAParSet : Inport  Description=Number of requested parameter set for Engine speed governor  OutMin=0  OutMax=255  OutDataTypeStr=State_uint8
  Constant : Constant  Value=ExtDem_Par0FacFdbkTrqLosHi_C
  Constant1 : Constant  Value=ExtDem_Par1FacFdbkTrqLosHi_C
  Constant2 : Constant  Value=ExtDem_Par2FacFdbkTrqLosHi_C
  Constant3 : Constant  Value=ExtDem_Par3FacFdbkTrqLosHi_C
  Constant4 : Constant  Value=ExtDem_Par4FacFdbkTrqLosHi_C
  Constant5 : Constant  Value=ExtDem_Par5FacFdbkTrqLosHi_C
  Constant6 : Constant  Value=ExtDem_Par6FacFdbkTrqLosHi_C
  Constant7 : Constant  Value=ExtDem_Par7FacFdbkTrqLosHi_C
  Multiport Switch1 : MultiPortSwitch  DataPortOrder=Zero-based contiguous  Inputs=8
  ExtDem_facFdbkTrqLosHi : Outport  Tag=rpm/Nm  Description=inner feedback factor for the upper setpoint  OutMin=-20  OutMax=20  OutDataTypeStr=FdbkNm2rpm_rpm_Nm
  wires:
  CoETS_numTSEAParSet/1 -> Multiport Switch1/1
  Multiport Switch1/1 -> ExtDem_facFdbkTrqLosHi/1
  Constant/1 -> Multiport Switch1/2
  Constant1/1 -> Multiport Switch1/3
  Constant2/1 -> Multiport Switch1/4
  Constant3/1 -> Multiport Switch1/5
  Constant4/1 -> Multiport Switch1/6
  Constant5/1 -> Multiport Switch1/7
  Constant6/1 -> Multiport Switch1/8
  Constant7/1 -> Multiport Switch1/9

== system ExtDem_SelectParameter/03_Feedback Factor / inner feedback factors /facFdbkTrqLosLo ==
  CoETS_numTSEAParSet : Inport  Description=Number of requested parameter set for Engine speed governor  OutMin=0  OutMax=255  OutDataTypeStr=State_uint8
  Constant : Constant  Value=ExtDem_Par0FacFdbkTrqLosLo_C
  Constant1 : Constant  Value=ExtDem_Par1FacFdbkTrqLosLo_C
  Constant2 : Constant  Value=ExtDem_Par2FacFdbkTrqLosLo_C
  Constant3 : Constant  Value=ExtDem_Par3FacFdbkTrqLosLo_C
  Constant4 : Constant  Value=ExtDem_Par4FacFdbkTrqLosLo_C
  Constant5 : Constant  Value=ExtDem_Par5FacFdbkTrqLosLo_C
  Constant6 : Constant  Value=ExtDem_Par6FacFdbkTrqLosLo_C
  Constant7 : Constant  Value=ExtDem_Par7FacFdbkTrqLosLo_C
  Multiport Switch1 : MultiPortSwitch  DataPortOrder=Zero-based contiguous  Inputs=8
  ExtDem_facFdbkTrqLosLo : Outport  Tag=rpm/Nm  Description=inner feedback factor for the lower setpoint  OutMin=-20  OutMax=20  OutDataTypeStr=FdbkNm2rpm_rpm_Nm
  wires:
  Multiport Switch1/1 -> ExtDem_facFdbkTrqLosLo/1
  Constant/1 -> Multiport Switch1/2
  Constant1/1 -> Multiport Switch1/3
  Constant2/1 -> Multiport Switch1/4
  Constant3/1 -> Multiport Switch1/5
  Constant4/1 -> Multiport Switch1/6
  Constant5/1 -> Multiport Switch1/7
  Constant6/1 -> Multiport Switch1/8
  Constant7/1 -> Multiport Switch1/9
  CoETS_numTSEAParSet/1 -> Multiport Switch1/1

== system ExtDem_SelectParameter/03_Feedback Factor / inner feedback factors /tiFltTrqLosEstCurr ==
  CoETS_numTSEAParSet : Inport  Description=Number of requested parameter set for Engine speed governor  OutMin=0  OutMax=255  OutDataTypeStr=State_uint8
  Constant : Constant  Value=ExtDem_Par0TiFltTrqLosEst_C
  Constant1 : Constant  Value=ExtDem_Par1TiFltTrqLosEst_C
  Constant2 : Constant  Value=ExtDem_Par2TiFltTrqLosEst_C
  Constant3 : Constant  Value=ExtDem_Par3TiFltTrqLosEst_C
  Constant4 : Constant  Value=ExtDem_Par4TiFltTrqLosEst_C
  Constant5 : Constant  Value=ExtDem_Par5TiFltTrqLosEst_C
  Constant6 : Constant  Value=ExtDem_Par6TiFltTrqLosEst_C
  Constant7 : Constant  Value=ExtDem_Par7TiFltTrqLosEst_C
  Multiport Switch1 : MultiPortSwitch  DataPortOrder=Zero-based contiguous  Inputs=8
  ExtDem_tiFltTrqLosEstCurr : Outport  Tag=s  Description=Time constant for EISGov torque loss calculation  OutMin=-180  OutMax=180  OutDataTypeStr=Time_s
  wires:
  CoETS_numTSEAParSet/1 -> Multiport Switch1/1
  Constant7/1 -> Multiport Switch1/9
  Constant6/1 -> Multiport Switch1/8
  Constant5/1 -> Multiport Switch1/7
  Constant4/1 -> Multiport Switch1/6
  Constant3/1 -> Multiport Switch1/5
  Constant2/1 -> Multiport Switch1/4
  Constant1/1 -> Multiport Switch1/3
  Constant/1 -> Multiport Switch1/2
  Multiport Switch1/1 -> ExtDem_tiFltTrqLosEstCurr/1

== system ExtDem_SelectParameter/03_Feedback Factor /outer feedback factor /ExtDem_ParXPKp_mp ==
  CoETS_numTSEAParSet : Inport  Description=Number of requested parameter set for Engine speed governor  OutMin=0  OutMax=255  OutDataTypeStr=State_uint8
  Constant1 : Constant  Value=ExtDem_facFdbkParSet0_C
  Constant2 : Constant  Value=ExtDem_facFdbkParSet1_C
  Constant3 : Constant  Value=ExtDem_facFdbkParSet2_C
  Constant4 : Constant  Value=ExtDem_facFdbkParSet3_C
  Constant5 : Constant  Value=ExtDem_facFdbkParSet4_C
  Constant6 : Constant  Value=ExtDem_facFdbkParSet5_C
  Constant7 : Constant  Value=ExtDem_facFdbkParSet6_C
  Constant8 : Constant  Value=ExtDem_facFdbkParSet7_C
  Multiport Switch1 : MultiPortSwitch  DataPortOrder=Zero-based contiguous  Inputs=8
  ExtDem_facFdbkParSet_mp : Outport
  wires:
  Constant1/1 -> Multiport Switch1/2
  Constant2/1 -> Multiport Switch1/3
  Constant3/1 -> Multiport Switch1/4
  Constant4/1 -> Multiport Switch1/5
  Constant5/1 -> Multiport Switch1/6
  Constant6/1 -> Multiport Switch1/7
  Constant7/1 -> Multiport Switch1/8
  Constant8/1 -> Multiport Switch1/9
  CoETS_numTSEAParSet/1 -> Multiport Switch1/1
  Multiport Switch1/1 -> ExtDem_facFdbkParSet_mp/1  "ExtDem_facFdbkParSet_mp"

== system ExtDem_SelectParameter/04_Limitation of the engine speed gradient /dnDecLim/ExtDem_stBrkTrq ==
  Brk_st : Inport  Description=Brake switch state  OutMin=0  OutMax=255  OutDataTypeStr=State_uint8
  CoETS_trqInrDesNTC : Inport  Tag=Nm  Description=Additional desired engine friction Nm  Port=2  OutMin=-3276  OutMax=3276  OutDataTypeStr=Trq_Nm
  Constant16 : Constant  Value=0  OutDataTypeStr=uint8
  Constant17 : Constant  Value=ExtDem_trqThresNTC_C
  Gain : Gain  Gain=2  OutDataTypeStr=uint8
  GetBit : CXLib/GetBit  dataTypeString=uint8  dataLength=0
      settings: AttributesFormatString=Get bit from %<dataTypeString>
  Relational Operator : RelationalOperator  Operator=<  OutDataTypeStr=boolean  RndMeth=Simplest
  Sum : Sum  Inputs=|++  OutDataTypeStr=uint8
  ExtDem_stBrkTrq_mp : Outport
  wires:
  Constant16/1 -> GetBit/2
  Brk_st/1 -> GetBit/1
  CoETS_trqInrDesNTC/1 -> Relational Operator/1
  Constant17/1 -> Relational Operator/2
  GetBit/1 -> Sum/1
  Relational Operator/1 -> Gain/1
  Gain/1 -> Sum/2
  Sum/1 -> ExtDem_stBrkTrq_mp/1
